simulink model "Sim_Multi"  (R2019b)
settings: Solver=VariableStepAuto  StartTime=0.0  StopTime=sim_time  FixedStep=t_sim  MaxStep=t_control  RelTol=1e-5  EnableMultiTasking=on
model workspace (MAT data in the model file):
  start_time = 1
values from neighbouring files (symbols this model uses):
  Att_init = [0;0;0] * d2r    [Init_Multi.m]
  Blade_flapping = 0    [Init_Multi.m]
  C_D = 0.40    (= 0.4)    [Init_Multi.m]
  CoG_nominal = [0;0;0.001]    [Init_Multi.m]
  CoG_real = [0;0;0.001]    [Init_Multi.m]
  Coriolis_correction = 0    [Init_Multi.m]
  d2r = pi/180    (= 0.0174532925199)    [Init_Multi.m]
  Dyn_thrust = 0    [Init_Multi.m]
  g = 9.80665    [Init_Multi.m]
  J_nominal = [Jxx Jxy Jxz;Jyx Jyy Jyz;Jzx Jzy Jzz]    [Init_Multi.m]
  J_real = [Jxx Jxy Jxz;Jyx Jyy Jyz;Jzx Jzy Jzz]    [Init_Multi.m]
  k1 = -1.125    [Init_Multi.m]
  k2 = -1.372    [Init_Multi.m]
  k3 = -1.718    [Init_Multi.m]
  k4 = -0.655    [Init_Multi.m]
  k_a1s = 1.5 / 4.0    (= 0.375)    [Init_Multi.m]
  k_beta = 0.23    [Init_Multi.m]
  kappa = 1.00    (= 1)    [Init_Multi.m]
  mass_nominal = 0.550    (= 0.55)    [Init_Multi.m]
  mass_real = 0.550    (= 0.55)    [Init_Multi.m]
  max_thrust = max_thrust + (MotorMatrix_nominal(i,7)*MotorMatrix_nominal(i,12)+MotorMatrix_nominal(i,8)*MotorMatrix_nominal(i,12)^2)    [Init_Multi.m]
  MaxRate_cmd = [360;360;120] * d2r    [Init_Multi.m]
  min_thrust = min_thrust + (MotorMatrix_nominal(i,7)*MotorMatrix_nominal(i,11)+MotorMatrix_nominal(i,8)*MotorMatrix_nominal(i,11)^2)    [Init_Multi.m]
  MotorMap = B' * inv(B * B')    [Init_Multi.m]
  MotorMatrix_nominal = [045 , 0.170 , -0.028 , -1 , 1.0 , 0.010 , [9.6820 , 0.010872]*1e-5 , [1.4504 , 0.0016312]*1e-6 , 0000 , 6000 , [0.0 , 0.0 , 0.0] , 8*2.54/100 , 11/1000;                         135 , 0.170 , -0.028 , +1 , 1.0 , 0.010 , [9.6820 , 0.010872]*1e-5 , [1.4504 , 0.0016312]*1e-6 , 0000 , 6000 , [0.0 , 0.0 , 0.0] , 8*2.54/100 , 11/1000;                         225 , 0.170 , -0.028 , -1 , 1.0 , 0.010 , [9. ...(+284 chars)    [Init_Multi.m]
  MotorMatrix_real = [045 , 0.170 , -0.028 , -1 , 1.0 , 0.010 , [9.6820 , 0.010872]*1e-5 , [1.4504 , 0.0016312]*1e-6 , 0000 , 6000 , [0.0 , 0.0 , 0.0] , 8*2.54/100 , 11/1000;                      135 , 0.170 , -0.028 , +1 , 1.0 , 0.010 , [9.6820 , 0.010872]*1e-5 , [1.4504 , 0.0016312]*1e-6 , 0000 , 6000 , [0.0 , 0.0 , 0.0] , 8*2.54/100 , 11/1000;                      225 , 0.170 , -0.028 , -1 , 1.0 , 0.010 , [9.6820 , ...(+275 chars)    [Init_Multi.m]
  Noise_flag = 1    [Init_Multi.m]
  omega_init = [0;0;0]    [Init_Multi.m]
  q_init = rpy2quat(Att_init)    [Init_Multi.m]
  r2d = 180/pi    (= 57.2957795131)    [Init_Multi.m]
  rho = 1.225    [Init_Multi.m]
  rpm2radpersec = 2*pi/60    (= 0.10471975512)    [Init_Multi.m]
  rpm_init = 3104.5025852    [Init_Multi.m]
  Surface_params = [a;b;c]    [Init_Multi.m]
  t_control = t_control_2*4    (= 0.02)    [Init_Multi.m]
  t_sim = 1/1000    (= 0.001)    [Init_Multi.m]
  thrust_reserve = 0.10    (= 0.1)    [Init_Multi.m]
  v_h = 4.0    (= 4)    [Init_Multi.m]
  Vb_init = [0;0;0]    [Init_Multi.m]
  Vi_init = R_IB_init' * Vb_init    [Init_Multi.m]
  Xi_init = [0;0;-1]    [Init_Multi.m]
undefined symbols (not defined in the file or in its folder): anti_windup_1, anti_windup_2, DiscIntNeverNeededParam, Kd_1, Kd_2, Kff_1, Kff_2, Ki_1, Ki_2, Kp_1, Kp_2, Kpass_1, magnitude, rpy2quat, thrust2rpm
libraries: simulink x35, dspsigops x3, sharedtransform x2, dspmtrx3 x1, robotuavlib x1, vrlib x1
(part 2 of 4)

== system Sim_Multi/State Estimation, Sensors, Noise/State estimation/Quat noise1 ==
  Band-Limited White Noise : simulink/Sources/Band-Limited White Noise  Cov=t_sim*57.3*57.3/10000  Ts=t_sim*30  seed=[23099]
  Constant : Constant  Value=Noise_flag
  Constant1 : Constant  Value=0
  Gain2 : Gain  Gain=0.1
  Rate Transition1 : RateTransition  OutPortSampleTime=t_sim
  Switch : Switch  Criteria=u2 > Threshold
  Noise : Outport
  wires:
  Band-Limited White Noise/1 -> Gain2/1
  Switch/1 -> Noise/1
  Constant/1 -> Switch/2
  Constant1/1 -> Switch/3
  Gain2/1 -> Rate Transition1/1
  Rate Transition1/1 -> Switch/1

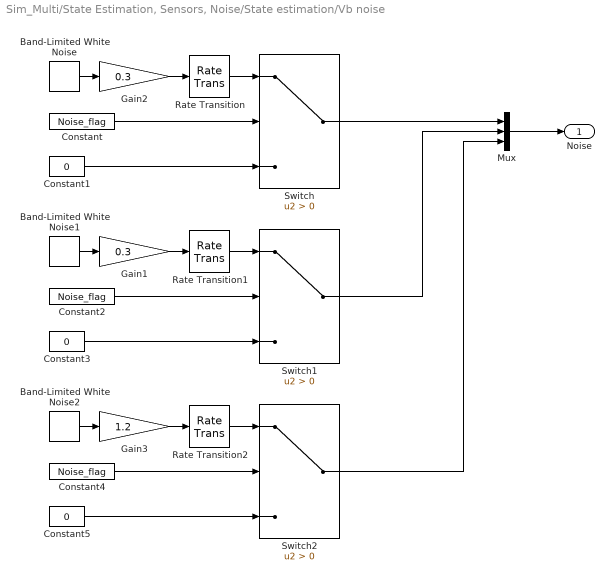
== system Sim_Multi/State Estimation, Sensors, Noise/State estimation/Vb noise ==
  Band-Limited White Noise : simulink/Sources/Band-Limited White Noise  Cov=t_sim*57.3*57.3/10000  Ts=t_sim*10  seed=[21234]
  Band-Limited White Noise1 : simulink/Sources/Band-Limited White Noise  Cov=t_sim*57.3*57.3/10000  Ts=t_sim*10  seed=[21234]
  Band-Limited White Noise2 : simulink/Sources/Band-Limited White Noise  Cov=t_sim*57.3*57.3/10000  Ts=t_sim*10  seed=[21234]
  Constant : Constant  Value=Noise_flag
  Constant1 : Constant  Value=0
  Constant2 : Constant  Value=Noise_flag
  Constant3 : Constant  Value=0
  Constant4 : Constant  Value=Noise_flag
  Constant5 : Constant  Value=0
  Gain1 : Gain  Gain=0.3
  Gain2 : Gain  Gain=0.3
  Gain3 : Gain  Gain=1.2
  Mux : Mux  Inputs=3
  Rate Transition : RateTransition  OutPortSampleTime=t_sim
  Rate Transition1 : RateTransition  OutPortSampleTime=t_sim
  Rate Transition2 : RateTransition  OutPortSampleTime=t_sim
  Switch : Switch  Criteria=u2 > Threshold
  Switch1 : Switch  Criteria=u2 > Threshold
  Switch2 : Switch  Criteria=u2 > Threshold
  Noise : Outport
  wires:
  Band-Limited White Noise/1 -> Gain2/1
  Constant/1 -> Switch/2
  Constant1/1 -> Switch/3
  Gain2/1 -> Rate Transition/1
  Rate Transition/1 -> Switch/1
  Switch/1 -> Mux/1
  Mux/1 -> Noise/1
  Band-Limited White Noise1/1 -> Gain1/1
  Constant2/1 -> Switch1/2
  Constant3/1 -> Switch1/3
  Gain1/1 -> Rate Transition1/1
  Rate Transition1/1 -> Switch1/1
  Band-Limited White Noise2/1 -> Gain3/1
  Constant4/1 -> Switch2/2
  Constant5/1 -> Switch2/3
  Gain3/1 -> Rate Transition2/1
  Rate Transition2/1 -> Switch2/1
  Switch1/1 -> Mux/2
  Switch2/1 -> Mux/3

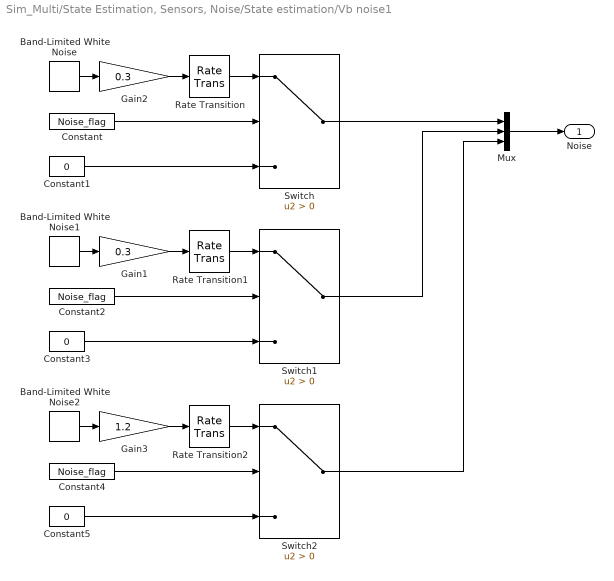
== system Sim_Multi/State Estimation, Sensors, Noise/State estimation/Vb noise1 ==
  Band-Limited White Noise : simulink/Sources/Band-Limited White Noise  Cov=t_sim*57.3*57.3/10000  Ts=t_sim*10  seed=[21234]
  Band-Limited White Noise1 : simulink/Sources/Band-Limited White Noise  Cov=t_sim*57.3*57.3/10000  Ts=t_sim*10  seed=[21234]
  Band-Limited White Noise2 : simulink/Sources/Band-Limited White Noise  Cov=t_sim*57.3*57.3/10000  Ts=t_sim*10  seed=[21234]
  Constant : Constant  Value=Noise_flag
  Constant1 : Constant  Value=0
  Constant2 : Constant  Value=Noise_flag
  Constant3 : Constant  Value=0
  Constant4 : Constant  Value=Noise_flag
  Constant5 : Constant  Value=0
  Gain1 : Gain  Gain=0.3
  Gain2 : Gain  Gain=0.3
  Gain3 : Gain  Gain=1.2
  Mux : Mux  Inputs=3
  Rate Transition : RateTransition  OutPortSampleTime=t_sim
  Rate Transition1 : RateTransition  OutPortSampleTime=t_sim
  Rate Transition2 : RateTransition  OutPortSampleTime=t_sim
  Switch : Switch  Criteria=u2 > Threshold
  Switch1 : Switch  Criteria=u2 > Threshold
  Switch2 : Switch  Criteria=u2 > Threshold
  Noise : Outport
  wires:
  Band-Limited White Noise/1 -> Gain2/1
  Constant/1 -> Switch/2
  Constant1/1 -> Switch/3
  Gain2/1 -> Rate Transition/1
  Rate Transition/1 -> Switch/1
  Switch/1 -> Mux/1
  Mux/1 -> Noise/1
  Band-Limited White Noise1/1 -> Gain1/1
  Constant2/1 -> Switch1/2
  Constant3/1 -> Switch1/3
  Gain1/1 -> Rate Transition1/1
  Rate Transition1/1 -> Switch1/1
  Band-Limited White Noise2/1 -> Gain3/1
  Constant4/1 -> Switch2/2
  Constant5/1 -> Switch2/3
  Gain3/1 -> Rate Transition2/1
  Rate Transition2/1 -> Switch2/1
  Switch1/1 -> Mux/2
  Switch2/1 -> Mux/3

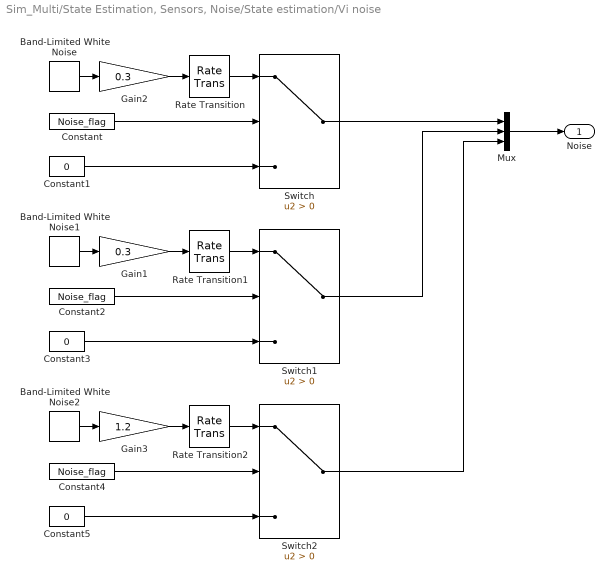
== system Sim_Multi/State Estimation, Sensors, Noise/State estimation/Vi noise ==
  Band-Limited White Noise : simulink/Sources/Band-Limited White Noise  Cov=t_sim*57.3*57.3/10000  Ts=t_sim*10  seed=[23888]
  Band-Limited White Noise1 : simulink/Sources/Band-Limited White Noise  Cov=t_sim*57.3*57.3/10000  Ts=t_sim*10  seed=[23888]
  Band-Limited White Noise2 : simulink/Sources/Band-Limited White Noise  Cov=t_sim*57.3*57.3/10000  Ts=t_sim*10  seed=[23888]
  Constant : Constant  Value=Noise_flag
  Constant1 : Constant  Value=0
  Constant2 : Constant  Value=Noise_flag
  Constant3 : Constant  Value=0
  Constant4 : Constant  Value=Noise_flag
  Constant5 : Constant  Value=0
  Gain1 : Gain  Gain=0.3
  Gain2 : Gain  Gain=0.3
  Gain3 : Gain  Gain=1.2
  Mux : Mux  Inputs=3
  Rate Transition : RateTransition  OutPortSampleTime=t_sim
  Rate Transition1 : RateTransition  OutPortSampleTime=t_sim
  Rate Transition2 : RateTransition  OutPortSampleTime=t_sim
  Switch : Switch  Criteria=u2 > Threshold
  Switch1 : Switch  Criteria=u2 > Threshold
  Switch2 : Switch  Criteria=u2 > Threshold
  Noise : Outport
  wires:
  Band-Limited White Noise/1 -> Gain2/1
  Constant/1 -> Switch/2
  Constant1/1 -> Switch/3
  Gain2/1 -> Rate Transition/1
  Rate Transition/1 -> Switch/1
  Switch/1 -> Mux/1
  Mux/1 -> Noise/1
  Band-Limited White Noise1/1 -> Gain1/1
  Constant2/1 -> Switch1/2
  Constant3/1 -> Switch1/3
  Gain1/1 -> Rate Transition1/1
  Rate Transition1/1 -> Switch1/1
  Band-Limited White Noise2/1 -> Gain3/1
  Constant4/1 -> Switch2/2
  Constant5/1 -> Switch2/3
  Gain3/1 -> Rate Transition2/1
  Rate Transition2/1 -> Switch2/1
  Switch1/1 -> Mux/2
  Switch2/1 -> Mux/3

== system Sim_Multi/State Estimation, Sensors, Noise/State estimation/Vi noise1 ==
  Band-Limited White Noise : simulink/Sources/Band-Limited White Noise  Cov=t_sim*57.3*57.3/10000  Ts=t_sim*10  seed=[23888]
  Band-Limited White Noise1 : simulink/Sources/Band-Limited White Noise  Cov=t_sim*57.3*57.3/10000  Ts=t_sim*10  seed=[23888]
  Band-Limited White Noise2 : simulink/Sources/Band-Limited White Noise  Cov=t_sim*57.3*57.3/10000  Ts=t_sim*10  seed=[23888]
  Constant : Constant  Value=Noise_flag
  Constant1 : Constant  Value=0
  Constant2 : Constant  Value=Noise_flag
  Constant3 : Constant  Value=0
  Constant4 : Constant  Value=Noise_flag
  Constant5 : Constant  Value=0
  Gain1 : Gain  Gain=0.3
  Gain2 : Gain  Gain=0.3
  Gain3 : Gain  Gain=1.2
  Mux : Mux  Inputs=3
  Rate Transition : RateTransition  OutPortSampleTime=t_sim
  Rate Transition1 : RateTransition  OutPortSampleTime=t_sim
  Rate Transition2 : RateTransition  OutPortSampleTime=t_sim
  Switch : Switch  Criteria=u2 > Threshold
  Switch1 : Switch  Criteria=u2 > Threshold
  Switch2 : Switch  Criteria=u2 > Threshold
  Noise : Outport
  wires:
  Band-Limited White Noise/1 -> Gain2/1
  Constant/1 -> Switch/2
  Constant1/1 -> Switch/3
  Gain2/1 -> Rate Transition/1
  Rate Transition/1 -> Switch/1
  Switch/1 -> Mux/1
  Mux/1 -> Noise/1
  Band-Limited White Noise1/1 -> Gain1/1
  Constant2/1 -> Switch1/2
  Constant3/1 -> Switch1/3
  Gain1/1 -> Rate Transition1/1
  Rate Transition1/1 -> Switch1/1
  Band-Limited White Noise2/1 -> Gain3/1
  Constant4/1 -> Switch2/2
  Constant5/1 -> Switch2/3
  Gain3/1 -> Rate Transition2/1
  Rate Transition2/1 -> Switch2/1
  Switch1/1 -> Mux/2
  Switch2/1 -> Mux/3

== system Sim_Multi/State Estimation, Sensors, Noise/State estimation/Xi noise ==
  Band-Limited White Noise : simulink/Sources/Band-Limited White Noise  Cov=t_sim*57.3*57.3/10000  Ts=t_sim*20  seed=[23559]
  Band-Limited White Noise1 : simulink/Sources/Band-Limited White Noise  Cov=t_sim*57.3*57.3/10000  Ts=t_sim*20  seed=[23559]
  Band-Limited White Noise2 : simulink/Sources/Band-Limited White Noise  Cov=t_sim*57.3*57.3/10000  Ts=t_sim*20  seed=[23559]
  Constant : Constant  Value=Noise_flag
  Constant1 : Constant  Value=0
  Constant2 : Constant  Value=Noise_flag
  Constant3 : Constant  Value=0
  Constant4 : Constant  Value=Noise_flag
  Constant5 : Constant  Value=0
  Gain1 : Gain  Gain=0.1
  Gain2 : Gain  Gain=0.1
  Gain3 : Gain  Gain=0.7
  Mux : Mux  Inputs=3
  Rate Transition : RateTransition  OutPortSampleTime=t_sim
  Rate Transition1 : RateTransition  OutPortSampleTime=t_sim
  Rate Transition2 : RateTransition  OutPortSampleTime=t_sim
  Switch : Switch  Criteria=u2 > Threshold
  Switch1 : Switch  Criteria=u2 > Threshold
  Switch2 : Switch  Criteria=u2 > Threshold
  Noise : Outport
  wires:
  Band-Limited White Noise/1 -> Gain2/1
  Constant/1 -> Switch/2
  Constant1/1 -> Switch/3
  Gain2/1 -> Rate Transition/1
  Mux/1 -> Noise/1
  Switch/1 -> Mux/1
  Band-Limited White Noise1/1 -> Gain1/1
  Constant2/1 -> Switch1/2
  Constant3/1 -> Switch1/3
  Gain1/1 -> Rate Transition1/1
  Band-Limited White Noise2/1 -> Gain3/1
  Constant4/1 -> Switch2/2
  Constant5/1 -> Switch2/3
  Gain3/1 -> Rate Transition2/1
  Switch1/1 -> Mux/2
  Switch2/1 -> Mux/3
  Rate Transition/1 -> Switch/1
  Rate Transition1/1 -> Switch1/1
  Rate Transition2/1 -> Switch2/1

== system Sim_Multi/State Estimation, Sensors, Noise/State estimation/Xi noise1 ==
  Band-Limited White Noise : simulink/Sources/Band-Limited White Noise  Cov=t_sim*57.3*57.3/10000  Ts=t_sim*20  seed=[23559]
  Band-Limited White Noise1 : simulink/Sources/Band-Limited White Noise  Cov=t_sim*57.3*57.3/10000  Ts=t_sim*20  seed=[23559]
  Band-Limited White Noise2 : simulink/Sources/Band-Limited White Noise  Cov=t_sim*57.3*57.3/10000  Ts=t_sim*20  seed=[23559]
  Constant : Constant  Value=Noise_flag
  Constant1 : Constant  Value=0
  Constant2 : Constant  Value=Noise_flag
  Constant3 : Constant  Value=0
  Constant4 : Constant  Value=Noise_flag
  Constant5 : Constant  Value=0
  Gain1 : Gain  Gain=0.1
  Gain2 : Gain  Gain=0.1
  Gain3 : Gain  Gain=0.7
  Mux : Mux  Inputs=3
  Rate Transition : RateTransition  OutPortSampleTime=t_sim
  Rate Transition1 : RateTransition  OutPortSampleTime=t_sim
  Rate Transition2 : RateTransition  OutPortSampleTime=t_sim
  Switch : Switch  Criteria=u2 > Threshold
  Switch1 : Switch  Criteria=u2 > Threshold
  Switch2 : Switch  Criteria=u2 > Threshold
  Noise : Outport
  wires:
  Band-Limited White Noise/1 -> Gain2/1
  Constant/1 -> Switch/2
  Constant1/1 -> Switch/3
  Gain2/1 -> Rate Transition/1
  Mux/1 -> Noise/1
  Switch/1 -> Mux/1
  Band-Limited White Noise1/1 -> Gain1/1
  Constant2/1 -> Switch1/2
  Constant3/1 -> Switch1/3
  Gain1/1 -> Rate Transition1/1
  Band-Limited White Noise2/1 -> Gain3/1
  Constant4/1 -> Switch2/2
  Constant5/1 -> Switch2/3
  Gain3/1 -> Rate Transition2/1
  Switch1/1 -> Mux/2
  Switch2/1 -> Mux/3
  Rate Transition/1 -> Switch/1
  Rate Transition1/1 -> Switch1/1
  Rate Transition2/1 -> Switch2/1

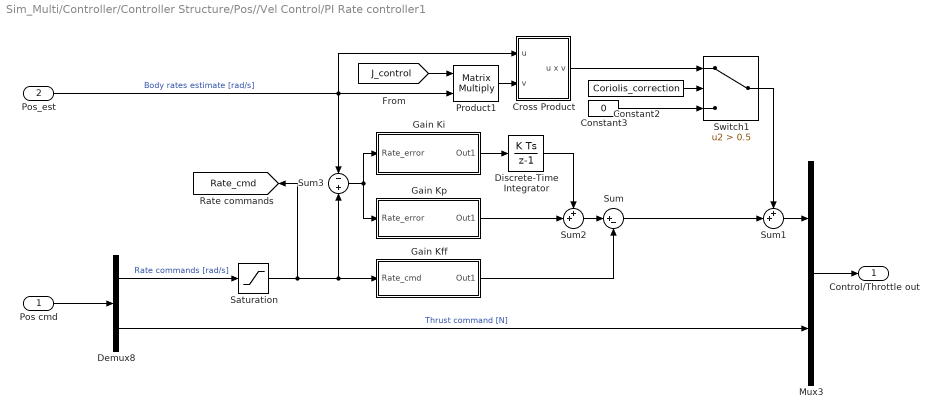
== system Sim_Multi/Controller/Controller Structure/Pos//Vel Control/PI Rate controller1 ==
  Pos cmd : Inport
  Pos_est : Inport  Port=2
  Constant2 : Constant  Value=Coriolis_correction
  Constant3 : Constant  Value=0
  Cross Product : Subsystem
  Demux8 : Demux  Outputs=[3 1]
  Discrete-Time Integrator : DiscreteIntegrator  SampleTime=t_control  ICPrevOutput=DiscIntNeverNeededParam  ICPrevScaledInput=DiscIntNeverNeededParam
  Gain Kff : Subsystem
  Gain Ki : Subsystem
  Gain Kp : Subsystem
  Mux3 : Mux  Inputs=2
  Product1 : Product  Multiplication=Matrix(*)  SampleTime=t_control  RndMeth=Zero
  Saturation : Saturate  UpperLimit=MaxRate_cmd  LowerLimit=-MaxRate_cmd
  Sum : Sum  Inputs=|+-
  Sum1 : Sum  Inputs=++|
  Sum2 : Sum  Inputs=++|
  Sum3 : Sum  Inputs=-|+
  Switch1 : Switch  Criteria=u2 > Threshold  Threshold=0.5  SampleTime=t_control
  Control/Throttle out : Outport
  tag scope: Rate_cmd=global
  wires:
  Pos_est/1 -> Product1/2, Sum3/1, Cross Product/1(u)  "Body rates estimate [rad/s]"
  Mux3/1 -> Control/Throttle out/1
  Pos cmd/1 -> Demux8/1
  Gain Ki/1(Out1) -> Discrete-Time Integrator/1
  Discrete-Time Integrator/1 -> Sum2/1
  Gain Kp/1(Out1) -> Sum2/2
  [J_control] -> Product1/1
  Product1/1 -> Cross Product/2(v)
  Sum1/1 -> Mux3/1
  Demux8/1 -> Saturation/1  "Rate commands [rad/s]"
  Sum3/1 -> Gain Kp/1(Rate_error), Gain Ki/1(Rate_error)
  Sum/1 -> Sum1/2
  Sum2/1 -> Sum/1
  Gain Kff/1(Out1) -> Sum/2
  Demux8/2 -> Mux3/2  "Thrust command [N]"
  Constant2/1 -> Switch1/2
  Cross Product/1(u x v) -> Switch1/1
  Constant3/1 -> Switch1/3
  Switch1/1 -> Sum1/1
  Saturation/1 -> [Rate_cmd], Sum3/2, Gain Kff/1(Rate_cmd)

== system Sim_Multi/Controller/Controller Structure/Pos//Vel Control/PID Attitude Controller (additionally controls altitude and yaw to take advantage of faster sampling rate)1 ==
  roll,pitch,yaw,Z_cmd : Inport
  roll,pitch,yaw,Z_est : Inport  Port=2
  Commands : Goto  Commented=on  GotoTag=rate_cmd  TagVisibility=global
  Constant : Constant  Value=Kff_2  SampleTime=-1
  Discrete Derivative : simulink/Discrete/Discrete Derivative  gainval=1.0  ICPrevScaledInput=0.0  OutMin=[]  OutMax=[]  OutDataType=fixdt(1, 16)  OutScaling=2^-10  DoSatur=off
  Discrete-Time Integrator : DiscreteIntegrator  SampleTime=-1  LimitOutput=on  UpperSaturationLimit=anti_windup_2  LowerSaturationLimit=-1*anti_windup_2  ICPrevOutput=DiscIntNeverNeededParam  ICPrevScaledInput=DiscIntNeverNeededParam
  Gain Kd : Subsystem
  Gain Ki : Subsystem
  Gain Kp : Subsystem
  Rate Transition : RateTransition  OutPortSampleTime=t_control_2
  Rate Transition1 : RateTransition  OutPortSampleTime=t_control_2
  Sum : Sum  Inputs=+++
  Sum2 : Sum  Inputs=++|
  Sum3 : Sum  Inputs=-|+
  Control/Velocity out : Outport
  wires:
  roll,pitch,yaw,Z_est/1 -> Rate Transition/1  "Body rates estimate [rad/s]"
  Sum/1 -> Control/Velocity out/1
  Gain Ki/1(Out1) -> Discrete-Time Integrator/1
  Discrete-Time Integrator/1 -> Sum2/1
  Gain Kp/1(Out1) -> Sum2/2
  Sum3/1 -> Gain Kp/1(Rate_error), Gain Ki/1(Rate_error)
  roll,pitch,yaw,Z_cmd/1 -> Rate Transition1/1
  Gain Kd/1(Out1) -> Sum/1
  Sum2/1 -> Sum/2
  Constant/1 -> Sum/3
  Discrete Derivative/1 -> Gain Kd/1(Rate_error)
  Rate Transition/1 -> Discrete Derivative/1, Sum3/1
  Rate Transition1/1 -> Commands/1, Sum3/2

== system Sim_Multi/Controller/Controller Structure/Pos//Vel Control/PID Attitude//Altitude Contorller ==
  roll,pitch,yaw,Z_cmd : Inport
  roll,pitch,yaw,Z_est : Inport  Port=2
  Constant : Constant  Value=5.4
  Demux : Demux
  Gain{,1..3} (4 alike) : Gain
  Mux : Mux
  PID Controller1 : simulink/Continuous/PID Controller  Controller=PID  Form=Parallel  TimeDomain=Discrete-time  SampleTime=-1  IntegratorMethod=Forward Euler  FilterMethod=Forward Euler  ControllerParametersSource=internal  P=0.061831432569432  I=0.0240439713230998  D=0.0379888953879029  UseFilter=on  N=83.1174994512611  TunerSelectOption=Transfer Function Based (PID Tuner App)  InitialConditionSource=internal  InitialConditionForIntegrator=0  InitialConditionForFilter=0  DifferentiatorICPrevScaledInput=0  ExternalReset=none  TrackingMode=off  Kt=1  LimitOutput=off  UpperSaturationLimit=inf  LowerSaturationLimit=-inf  LinearizeAsGain=on  AntiWindupMode=none  Kb=1  POutMin=[]  POutMax=[]  IOutMin=[]  IOutMax=[]  DOutMin=[]  DOutMax=[]  NOutMin=[]  NOutMax=[]  SumOutMin=[]  SumOutMax=[]  SaturationOutMin=[]  SaturationOutMax=[]  PParamMin=[]  PParamMax=[]  IParamMin=[]  IParamMax=[]  DParamMin=[]  DParamMax=[]  NParamMin=[]  NParamMax=[]  KbParamMin=[]  KbParamMax=[]  KtParamMin=[]  KtParamMax=[]  KbOutMin=[]  KbOutMax=[]  KtOutMin=[]  KtOutMax=[]  IntegratorOutMin=[]  IntegratorOutMax=[]  FilterOutMin=[]  FilterOutMax=[]  SumI1OutMin=[]  SumI1OutMax=[]  SumI2OutMin=[]  SumI2OutMax=[]  SumI3OutMin=[]  SumI3OutMax=[]  SumI4OutMin=[]  SumI4OutMax=[]  SumDOutMin=[]  SumDOutMax=[]  DifferentiatorOutMin=[]  DifferentiatorOutMax=[]  FilterDiffOutCoefMin=[]  FilterDiffOutCoefMax=[]  ReciprocalOutMin=[]  ReciprocalOutMax=[]  SumDenOutMin=[]  SumDenOutMax=[]  SumNumOutMin=[]  SumNumOutMax=[]  DivideOutMin=[]  DivideOutMax=[]  IntegratorContinuousStateAttributes=''  IntegratorStateMustResolveToSignalObject=off  IntegratorRTWStateStorageClass=Auto  FilterContinuousStateAttributes=''  FilterStateMustResolveToSignalObject=off  FilterRTWStateStorageClass=Auto  ParallelPVariant=InternalParameters  IdealPVariant=Disabled  IVariant=InternalParameters  DVariant=InternalParameters  IntegratorVariant=Discrete  SatVariant=Disabled  AWVariant=Passthrough  PCopyVariant=Disabled  TRVariant=Disabled  FdbkBlocksVariant=Forward  IdealPFdbkVariant=Disabled  SatFdbkVariant=Disabled  DerivativeFilterVariant=ForwardEulerFilter  NVariant=InternalParameters  NCopyVariant=Disabled  FilterICVariant=InternalICsFilter  IntegratorICVariant=InternalICs  ExternalResetVariant=Disabled  TRSumVariant=Passthrough  SumFdbkVariant=Disabled  SumVariant=Sum_PID
  PID Controller2 : simulink/Continuous/PID Controller  Controller=PID  Form=Parallel  TimeDomain=Discrete-time  SampleTime=-1  IntegratorMethod=Forward Euler  FilterMethod=Forward Euler  ControllerParametersSource=internal  P=0.00183714357509643  I=9.47923809923689e-05  D=0.00707292143048776  UseFilter=on  N=10.221680571317  TunerSelectOption=Transfer Function Based (PID Tuner App)  InitialConditionSource=internal  InitialConditionForIntegrator=0  InitialConditionForFilter=0  DifferentiatorICPrevScaledInput=0  ExternalReset=none  TrackingMode=off  Kt=1  LimitOutput=off  UpperSaturationLimit=inf  LowerSaturationLimit=-inf  LinearizeAsGain=on  AntiWindupMode=none  Kb=1  POutMin=[]  POutMax=[]  IOutMin=[]  IOutMax=[]  DOutMin=[]  DOutMax=[]  NOutMin=[]  NOutMax=[]  SumOutMin=[]  SumOutMax=[]  SaturationOutMin=[]  SaturationOutMax=[]  PParamMin=[]  PParamMax=[]  IParamMin=[]  IParamMax=[]  DParamMin=[]  DParamMax=[]  NParamMin=[]  NParamMax=[]  KbParamMin=[]  KbParamMax=[]  KtParamMin=[]  KtParamMax=[]  KbOutMin=[]  KbOutMax=[]  KtOutMin=[]  KtOutMax=[]  IntegratorOutMin=[]  IntegratorOutMax=[]  FilterOutMin=[]  FilterOutMax=[]  SumI1OutMin=[]  SumI1OutMax=[]  SumI2OutMin=[]  SumI2OutMax=[]  SumI3OutMin=[]  SumI3OutMax=[]  SumI4OutMin=[]  SumI4OutMax=[]  SumDOutMin=[]  SumDOutMax=[]  DifferentiatorOutMin=[]  DifferentiatorOutMax=[]  FilterDiffOutCoefMin=[]  FilterDiffOutCoefMax=[]  ReciprocalOutMin=[]  ReciprocalOutMax=[]  SumDenOutMin=[]  SumDenOutMax=[]  SumNumOutMin=[]  SumNumOutMax=[]  DivideOutMin=[]  DivideOutMax=[]  IntegratorContinuousStateAttributes=''  IntegratorStateMustResolveToSignalObject=off  IntegratorRTWStateStorageClass=Auto  FilterContinuousStateAttributes=''  FilterStateMustResolveToSignalObject=off  FilterRTWStateStorageClass=Auto  ParallelPVariant=InternalParameters  IdealPVariant=Disabled  IVariant=InternalParameters  DVariant=InternalParameters  IntegratorVariant=Discrete  SatVariant=Disabled  AWVariant=Passthrough  PCopyVariant=Disabled  TRVariant=Disabled  FdbkBlocksVariant=Forward  IdealPFdbkVariant=Disabled  SatFdbkVariant=Disabled  DerivativeFilterVariant=ForwardEulerFilter  NVariant=InternalParameters  NCopyVariant=Disabled  FilterICVariant=InternalICsFilter  IntegratorICVariant=InternalICs  ExternalResetVariant=Disabled  TRSumVariant=Passthrough  SumFdbkVariant=Disabled  SumVariant=Sum_PID
  PID Controller3 : simulink/Continuous/PID Controller  Controller=PID  Form=Parallel  TimeDomain=Discrete-time  SampleTime=-1  IntegratorMethod=Forward Euler  FilterMethod=Forward Euler  ControllerParametersSource=internal  P=-0.137480258273751  I=-0.00709366496874399  D=-0.529292907856896  UseFilter=on  N=10.221680571317  TunerSelectOption=Transfer Function Based (PID Tuner App)  InitialConditionSource=internal  InitialConditionForIntegrator=0  InitialConditionForFilter=0  DifferentiatorICPrevScaledInput=0  ExternalReset=none  TrackingMode=off  Kt=1  LimitOutput=off  UpperSaturationLimit=inf  LowerSaturationLimit=-inf  LinearizeAsGain=on  AntiWindupMode=none  Kb=1  POutMin=[]  POutMax=[]  IOutMin=[]  IOutMax=[]  DOutMin=[]  DOutMax=[]  NOutMin=[]  NOutMax=[]  SumOutMin=[]  SumOutMax=[]  SaturationOutMin=[]  SaturationOutMax=[]  PParamMin=[]  PParamMax=[]  IParamMin=[]  IParamMax=[]  DParamMin=[]  DParamMax=[]  NParamMin=[]  NParamMax=[]  KbParamMin=[]  KbParamMax=[]  KtParamMin=[]  KtParamMax=[]  KbOutMin=[]  KbOutMax=[]  KtOutMin=[]  KtOutMax=[]  IntegratorOutMin=[]  IntegratorOutMax=[]  FilterOutMin=[]  FilterOutMax=[]  SumI1OutMin=[]  SumI1OutMax=[]  SumI2OutMin=[]  SumI2OutMax=[]  SumI3OutMin=[]  SumI3OutMax=[]  SumI4OutMin=[]  SumI4OutMax=[]  SumDOutMin=[]  SumDOutMax=[]  DifferentiatorOutMin=[]  DifferentiatorOutMax=[]  FilterDiffOutCoefMin=[]  FilterDiffOutCoefMax=[]  ReciprocalOutMin=[]  ReciprocalOutMax=[]  SumDenOutMin=[]  SumDenOutMax=[]  SumNumOutMin=[]  SumNumOutMax=[]  DivideOutMin=[]  DivideOutMax=[]  IntegratorContinuousStateAttributes=''  IntegratorStateMustResolveToSignalObject=off  IntegratorRTWStateStorageClass=Auto  FilterContinuousStateAttributes=''  FilterStateMustResolveToSignalObject=off  FilterRTWStateStorageClass=Auto  ParallelPVariant=InternalParameters  IdealPVariant=Disabled  IVariant=InternalParameters  DVariant=InternalParameters  IntegratorVariant=Discrete  SatVariant=Disabled  AWVariant=Passthrough  PCopyVariant=Disabled  TRVariant=Disabled  FdbkBlocksVariant=Forward  IdealPFdbkVariant=Disabled  SatFdbkVariant=Disabled  DerivativeFilterVariant=ForwardEulerFilter  NVariant=InternalParameters  NCopyVariant=Disabled  FilterICVariant=InternalICsFilter  IntegratorICVariant=InternalICs  ExternalResetVariant=Disabled  TRSumVariant=Passthrough  SumFdbkVariant=Disabled  SumVariant=Sum_PID
  PID Controller4 : simulink/Continuous/PID Controller  Controller=PID  Form=Parallel  TimeDomain=Discrete-time  SampleTime=-1  IntegratorMethod=Forward Euler  FilterMethod=Forward Euler  ControllerParametersSource=internal  P=0.0636807472008284  I=0.0247631018062204  D=0.0391251042246079  UseFilter=on  N=83.1174994512611  TunerSelectOption=Transfer Function Based (PID Tuner App)  InitialConditionSource=internal  InitialConditionForIntegrator=0  InitialConditionForFilter=0  DifferentiatorICPrevScaledInput=0  ExternalReset=none  TrackingMode=off  Kt=1  LimitOutput=off  UpperSaturationLimit=inf  LowerSaturationLimit=-inf  LinearizeAsGain=on  AntiWindupMode=none  Kb=1  POutMin=[]  POutMax=[]  IOutMin=[]  IOutMax=[]  DOutMin=[]  DOutMax=[]  NOutMin=[]  NOutMax=[]  SumOutMin=[]  SumOutMax=[]  SaturationOutMin=[]  SaturationOutMax=[]  PParamMin=[]  PParamMax=[]  IParamMin=[]  IParamMax=[]  DParamMin=[]  DParamMax=[]  NParamMin=[]  NParamMax=[]  KbParamMin=[]  KbParamMax=[]  KtParamMin=[]  KtParamMax=[]  KbOutMin=[]  KbOutMax=[]  KtOutMin=[]  KtOutMax=[]  IntegratorOutMin=[]  IntegratorOutMax=[]  FilterOutMin=[]  FilterOutMax=[]  SumI1OutMin=[]  SumI1OutMax=[]  SumI2OutMin=[]  SumI2OutMax=[]  SumI3OutMin=[]  SumI3OutMax=[]  SumI4OutMin=[]  SumI4OutMax=[]  SumDOutMin=[]  SumDOutMax=[]  DifferentiatorOutMin=[]  DifferentiatorOutMax=[]  FilterDiffOutCoefMin=[]  FilterDiffOutCoefMax=[]  ReciprocalOutMin=[]  ReciprocalOutMax=[]  SumDenOutMin=[]  SumDenOutMax=[]  SumNumOutMin=[]  SumNumOutMax=[]  DivideOutMin=[]  DivideOutMax=[]  IntegratorContinuousStateAttributes=''  IntegratorStateMustResolveToSignalObject=off  IntegratorRTWStateStorageClass=Auto  FilterContinuousStateAttributes=''  FilterStateMustResolveToSignalObject=off  FilterRTWStateStorageClass=Auto  ParallelPVariant=InternalParameters  IdealPVariant=Disabled  IVariant=InternalParameters  DVariant=InternalParameters  IntegratorVariant=Discrete  SatVariant=Disabled  AWVariant=Passthrough  PCopyVariant=Disabled  TRVariant=Disabled  FdbkBlocksVariant=Forward  IdealPFdbkVariant=Disabled  SatFdbkVariant=Disabled  DerivativeFilterVariant=ForwardEulerFilter  NVariant=InternalParameters  NCopyVariant=Disabled  FilterICVariant=InternalICsFilter  IntegratorICVariant=InternalICs  ExternalResetVariant=Disabled  TRSumVariant=Passthrough  SumFdbkVariant=Disabled  SumVariant=Sum_PID
  Rate Transition1 : RateTransition  OutPortSampleTime=t_control_2
  Rate Transition2 : RateTransition  OutPortSampleTime=t_control_2
  Scope3 : Scope  NumInputPorts=4
  Sum : Sum  Inputs=|++
  Sum3 : Sum  Inputs=-|+
  Control/Velocity out : Outport
  wires:
  PID Controller3/1 -> Gain3/1
  PID Controller1/1 -> Gain1/1
  Gain/1 -> Mux/1
  roll,pitch,yaw,Z_cmd/1 -> Rate Transition1/1
  Gain2/1 -> Mux/3
  Sum3/1 -> Demux/1
  Mux/1 -> Rate Transition2/1
  Sum/1 -> Mux/4
  PID Controller2/1 -> Gain2/1
  Gain3/1 -> Sum/1
  Constant/1 -> Sum/2
  PID Controller4/1 -> Gain/1
  roll,pitch,yaw,Z_est/1 -> Sum3/1
  Gain1/1 -> Mux/2
  Demux/2 -> Scope3/2, PID Controller1/1
  Rate Transition1/1 -> Sum3/2
  Demux/4 -> Scope3/4, PID Controller3/1
  Demux/3 -> Scope3/3, PID Controller2/1
  Demux/1 -> Scope3/1, PID Controller4/1
  Rate Transition2/1 -> Control/Velocity out/1

== system Sim_Multi/Controller/Controller Structure/Pos//Vel Control/PID Position Controller (yaw and Z are passed though) ==
  (Y,X,yaw,Z)_cmd : Inport
  (Y,X,yaw,Z)_est : Inport  Port=2
  Demux : Demux
  Demux1 : Demux
  Gain : Gain
  Gain1 : Gain
  Mux : Mux
  PID Controller1 : simulink/Continuous/PID Controller  Controller=PID  Form=Parallel  TimeDomain=Discrete-time  SampleTime=-1  IntegratorMethod=Forward Euler  FilterMethod=Forward Euler  ControllerParametersSource=internal  P=-0.0202827380782485  I=-0.00081616740602595  D=-0.0881024693027783  UseFilter=on  N=9.03936793379723  TunerSelectOption=Transfer Function Based (PID Tuner App)  InitialConditionSource=internal  InitialConditionForIntegrator=0  InitialConditionForFilter=0  DifferentiatorICPrevScaledInput=0  ExternalReset=none  TrackingMode=off  Kt=1  LimitOutput=off  UpperSaturationLimit=inf  LowerSaturationLimit=-inf  LinearizeAsGain=on  AntiWindupMode=none  Kb=1  POutMin=[]  POutMax=[]  IOutMin=[]  IOutMax=[]  DOutMin=[]  DOutMax=[]  NOutMin=[]  NOutMax=[]  SumOutMin=[]  SumOutMax=[]  SaturationOutMin=[]  SaturationOutMax=[]  PParamMin=[]  PParamMax=[]  IParamMin=[]  IParamMax=[]  DParamMin=[]  DParamMax=[]  NParamMin=[]  NParamMax=[]  KbParamMin=[]  KbParamMax=[]  KtParamMin=[]  KtParamMax=[]  KbOutMin=[]  KbOutMax=[]  KtOutMin=[]  KtOutMax=[]  IntegratorOutMin=[]  IntegratorOutMax=[]  FilterOutMin=[]  FilterOutMax=[]  SumI1OutMin=[]  SumI1OutMax=[]  SumI2OutMin=[]  SumI2OutMax=[]  SumI3OutMin=[]  SumI3OutMax=[]  SumI4OutMin=[]  SumI4OutMax=[]  SumDOutMin=[]  SumDOutMax=[]  DifferentiatorOutMin=[]  DifferentiatorOutMax=[]  FilterDiffOutCoefMin=[]  FilterDiffOutCoefMax=[]  ReciprocalOutMin=[]  ReciprocalOutMax=[]  SumDenOutMin=[]  SumDenOutMax=[]  SumNumOutMin=[]  SumNumOutMax=[]  DivideOutMin=[]  DivideOutMax=[]  IntegratorContinuousStateAttributes=''  IntegratorStateMustResolveToSignalObject=off  IntegratorRTWStateStorageClass=Auto  FilterContinuousStateAttributes=''  FilterStateMustResolveToSignalObject=off  FilterRTWStateStorageClass=Auto  ParallelPVariant=InternalParameters  IdealPVariant=Disabled  IVariant=InternalParameters  DVariant=InternalParameters  IntegratorVariant=Discrete  SatVariant=Disabled  AWVariant=Passthrough  PCopyVariant=Disabled  TRVariant=Disabled  FdbkBlocksVariant=Forward  IdealPFdbkVariant=Disabled  SatFdbkVariant=Disabled  DerivativeFilterVariant=ForwardEulerFilter  NVariant=InternalParameters  NCopyVariant=Disabled  FilterICVariant=InternalICsFilter  IntegratorICVariant=InternalICs  ExternalResetVariant=Disabled  TRSumVariant=Passthrough  SumFdbkVariant=Disabled  SumVariant=Sum_PID
  PID Controller4 : simulink/Continuous/PID Controller  Controller=PID  Form=Parallel  TimeDomain=Discrete-time  SampleTime=-1  IntegratorMethod=Forward Euler  FilterMethod=Forward Euler  ControllerParametersSource=internal  P=0.0202827380772714  I=0.000816167405912946  D=0.0881024692983823  UseFilter=on  N=9.03936793379723  TunerSelectOption=Transfer Function Based (PID Tuner App)  InitialConditionSource=internal  InitialConditionForIntegrator=0  InitialConditionForFilter=0  DifferentiatorICPrevScaledInput=0  ExternalReset=none  TrackingMode=off  Kt=1  LimitOutput=off  UpperSaturationLimit=inf  LowerSaturationLimit=-inf  LinearizeAsGain=on  AntiWindupMode=none  Kb=1  POutMin=[]  POutMax=[]  IOutMin=[]  IOutMax=[]  DOutMin=[]  DOutMax=[]  NOutMin=[]  NOutMax=[]  SumOutMin=[]  SumOutMax=[]  SaturationOutMin=[]  SaturationOutMax=[]  PParamMin=[]  PParamMax=[]  IParamMin=[]  IParamMax=[]  DParamMin=[]  DParamMax=[]  NParamMin=[]  NParamMax=[]  KbParamMin=[]  KbParamMax=[]  KtParamMin=[]  KtParamMax=[]  KbOutMin=[]  KbOutMax=[]  KtOutMin=[]  KtOutMax=[]  IntegratorOutMin=[]  IntegratorOutMax=[]  FilterOutMin=[]  FilterOutMax=[]  SumI1OutMin=[]  SumI1OutMax=[]  SumI2OutMin=[]  SumI2OutMax=[]  SumI3OutMin=[]  SumI3OutMax=[]  SumI4OutMin=[]  SumI4OutMax=[]  SumDOutMin=[]  SumDOutMax=[]  DifferentiatorOutMin=[]  DifferentiatorOutMax=[]  FilterDiffOutCoefMin=[]  FilterDiffOutCoefMax=[]  ReciprocalOutMin=[]  ReciprocalOutMax=[]  SumDenOutMin=[]  SumDenOutMax=[]  SumNumOutMin=[]  SumNumOutMax=[]  DivideOutMin=[]  DivideOutMax=[]  IntegratorContinuousStateAttributes=''  IntegratorStateMustResolveToSignalObject=off  IntegratorRTWStateStorageClass=Auto  FilterContinuousStateAttributes=''  FilterStateMustResolveToSignalObject=off  FilterRTWStateStorageClass=Auto  ParallelPVariant=InternalParameters  IdealPVariant=Disabled  IVariant=InternalParameters  DVariant=InternalParameters  IntegratorVariant=Discrete  SatVariant=Disabled  AWVariant=Passthrough  PCopyVariant=Disabled  TRVariant=Disabled  FdbkBlocksVariant=Forward  IdealPFdbkVariant=Disabled  SatFdbkVariant=Disabled  DerivativeFilterVariant=ForwardEulerFilter  NVariant=InternalParameters  NCopyVariant=Disabled  FilterICVariant=InternalICsFilter  IntegratorICVariant=InternalICs  ExternalResetVariant=Disabled  TRSumVariant=Passthrough  SumFdbkVariant=Disabled  SumVariant=Sum_PID
  Rate Transition : RateTransition  Integrity=off  OutPortSampleTime=t_control
  Rate Transition1 : RateTransition  Integrity=off  OutPortSampleTime=t_control
  Scope3 : Scope  NumInputPorts=2
  Sum3 : Sum  Inputs=-|+
  Terminator{,1..3} (4 alike) : Terminator
  roll,pitch,yaw,climb cmd : Outport
  tag scope: cmd=global
  wires:
  (Y,X,yaw,Z)_est/1 -> Rate Transition/1
  (Y,X,yaw,Z)_cmd/1 -> Rate Transition1/1
  Rate Transition1/1 -> Demux1/1, Sum3/2, [cmd]
  Rate Transition/1 -> Sum3/1
  Demux/2 -> Scope3/2, PID Controller1/1
  Gain1/1 -> Mux/2
  PID Controller4/1 -> Gain/1
  Sum3/1 -> Demux/1
  PID Controller1/1 -> Gain1/1
  Mux/1 -> roll,pitch,yaw,climb cmd/1
  Gain/1 -> Mux/1
  Demux/1 -> Scope3/1, PID Controller4/1
  Demux/3 -> Terminator/1
  Demux/4 -> Terminator1/1
  Demux1/4 -> Mux/4
  Demux1/3 -> Mux/3
  Demux1/1 -> Terminator2/1
  Demux1/2 -> Terminator3/1

== system Sim_Multi/Controller/Controller Structure/Pos//Vel Control/PID Position Controller (yaw and Z are passed though)1 ==
  (Y,X,yaw,Z)_cmd : Inport
  (Y,X,yaw,Z)_est : Inport  Port=2
  Constant : Constant  Value=Kff_1  SampleTime=t_control
  Discrete Derivative : simulink/Discrete/Discrete Derivative  gainval=1.0  ICPrevScaledInput=0.0  OutMin=[]  OutMax=[]  OutDataType=fixdt(1, 16)  OutScaling=2^-10  DoSatur=off
  Discrete-Time Integrator : DiscreteIntegrator  SampleTime=t_control  LimitOutput=on  UpperSaturationLimit=anti_windup_1  LowerSaturationLimit=-1*anti_windup_1  ICPrevOutput=DiscIntNeverNeededParam  ICPrevScaledInput=DiscIntNeverNeededParam
  Gain : Gain  Gain=Kpass_1
  Gain Kd : Subsystem
  Gain Ki : Subsystem
  Gain Kp : Subsystem
  Rate Transition : RateTransition  OutPortSampleTime=t_control
  Rate Transition1 : RateTransition  OutPortSampleTime=t_control
  Sum : Sum  Inputs=+++
  Sum2 : Sum  Inputs=+++
  Sum3 : Sum  Inputs=-|+
  roll,pitch,yaw,climb cmd : Outport
  tag scope: cmd=global
  wires:
  (Y,X,yaw,Z)_est/1 -> Rate Transition/1
  Sum/1 -> roll,pitch,yaw,climb cmd/1
  Gain Ki/1(Out1) -> Discrete-Time Integrator/1
  Discrete-Time Integrator/1 -> Sum2/1
  Gain Kp/1(Out1) -> Sum2/2
  Sum3/1 -> Gain Kp/1(Rate_error), Gain Ki/1(Rate_error)
  (Y,X,yaw,Z)_cmd/1 -> Rate Transition1/1
  Gain Kd/1(Out1) -> Sum/1
  Sum2/1 -> Sum/2
  Constant/1 -> Sum/3
  Discrete Derivative/1 -> Gain Kd/1(Rate_error)
  Rate Transition1/1 -> [cmd], Gain/1, Sum3/2
  Rate Transition/1 -> Discrete Derivative/1, Sum3/1
  Gain/1 -> Sum2/3

== system Sim_Multi/Plant/6DOF model/Calculate omega_dot/Cross Product omega x (J * omega) ==
  omega : Inport
  J * omega : Inport  Port=2
  Subsystem : Subsystem
  Subsystem1 : Subsystem
  Sum : Sum  Inputs=+|-
  omega x (J * omega) : Outport
  wires:
  Sum/1 -> omega x (J * omega)/1
  omega/1 -> Subsystem1/1(u), Subsystem/1(u)
  J * omega/1 -> Subsystem/2(v), Subsystem1/2(v)
  Subsystem/1(Positive elements) -> Sum/1
  Subsystem1/1(Negative elements) -> Sum/2

== system Sim_Multi/Plant/6DOF model/Calculate omega_dot/Subsystem ==
  omega : Inport
  J : Inport  Port=2
  Product : Product  Multiplication=Matrix(*)
  Reshape : Reshape  OutputDimensionality=Column vector (2-D)
  Reshape1 : Reshape  OutputDimensionality=Column vector (2-D)
  J * omega : Outport
  wires:
  Reshape1/1 -> J * omega/1
  Product/1 -> Reshape1/1
  J/1 -> Product/1
  Reshape/1 -> Product/2
  omega/1 -> Reshape/1

== system Sim_Multi/Plant/6DOF model/Quat Strapdown Eq./Cross Product ==
  u : Inport
  v : Inport  Port=2
  Subsystem : Subsystem
  Subsystem1 : Subsystem
  Sum : Sum  Inputs=+|-
  u x v : Outport
  wires:
  Sum/1 -> u x v/1
  u/1 -> Subsystem1/1(u), Subsystem/1(u)
  v/1 -> Subsystem1/2(v), Subsystem/2(v)
  Subsystem/1(Positive elements) -> Sum/1
  Subsystem1/1(Negative elements) -> Sum/2

== system Sim_Multi/Plant/6DOF model/Quat Strapdown Eq./Dot product ==
  u : Inport
  v : Inport  Port=2
  Product : Product  Multiplication=Matrix(*)  RndMeth=Zero
  Reshape : Reshape  OutputDimensionality=Column vector (2-D)
  Reshape1 : Reshape  OutputDimensionality=Column vector (2-D)
  transpose : Math  Operator=transpose  SaturateOnIntegerOverflow=on
  u.v : Outport
  wires:
  v/1 -> Reshape1/1
  u/1 -> Reshape/1
  Reshape/1 -> transpose/1
  transpose/1 -> Product/1
  Reshape1/1 -> Product/2
  Product/1 -> u.v/1

== system Sim_Multi/Plant/6DOF model/Quat Strapdown Eq./Normalize ==
  Input : Inport
  Divide : Product  Inputs=*/
  norm : Subsystem
  Output : Outport
  wires:
  Input/1 -> Divide/1, norm/1(u)
  norm/1(||u||) -> Divide/2
  Divide/1 -> Output/1

== system Sim_Multi/Plant/6DOF model/Quat to Rotation Matrix/Subsystem ==
  q : Inport
  Add : Sum  Inputs=++--
  Demux : Demux
  Product{,2..4} (4 alike) : Product
  C_11 : Outport
  wires:
  Product2/1 -> Add/2
  Product4/1 -> Add/4
  Add/1 -> C_11/1
  Demux/2 -> Product2/2, Product2/1
  Product3/1 -> Add/3
  Demux/3 -> Product3/2, Product3/1
  Demux/1 -> Product/2, Product/1
  q/1 -> Demux/1
  Product/1 -> Add/1
  Demux/4 -> Product4/2, Product4/1

== system Sim_Multi/Plant/6DOF model/Quat to Rotation Matrix/Subsystem1 ==
  q : Inport
  Add : Sum  Inputs=+-+-
  Demux : Demux
  Product{,2..4} (4 alike) : Product
  C_22 : Outport
  wires:
  Product2/1 -> Add/2
  Product4/1 -> Add/4
  Add/1 -> C_22/1
  Demux/2 -> Product2/2, Product2/1
  Product3/1 -> Add/3
  Demux/3 -> Product3/2, Product3/1
  Demux/1 -> Product/2, Product/1
  q/1 -> Demux/1
  Product/1 -> Add/1
  Demux/4 -> Product4/2, Product4/1

== system Sim_Multi/Plant/6DOF model/Quat to Rotation Matrix/Subsystem2 ==
  q : Inport
  Add : Sum  Inputs=+--+
  Demux : Demux
  Product{,2..4} (4 alike) : Product
  C_33 : Outport
  wires:
  Product2/1 -> Add/2
  Product4/1 -> Add/4
  Add/1 -> C_33/1
  Demux/2 -> Product2/2, Product2/1
  Product3/1 -> Add/3
  Demux/3 -> Product3/2, Product3/1
  Demux/1 -> Product/2, Product/1
  q/1 -> Demux/1
  Product/1 -> Add/1
  Demux/4 -> Product4/2, Product4/1

== system Sim_Multi/Plant/6DOF model/Quat to Rotation Matrix/Subsystem3 ==
  q : Inport
  Add : Sum
  Demux : Demux
  Gain : Gain  Gain=2
  Product : Product
  Product2 : Product
  C_12 : Outport
  wires:
  Add/1 -> Gain/1
  q/1 -> Demux/1
  Demux/2 -> Product/1
  Demux/3 -> Product/2
  Demux/1 -> Product2/1
  Demux/4 -> Product2/2
  Product/1 -> Add/1
  Product2/1 -> Add/2
  Gain/1 -> C_12/1

== system Sim_Multi/Plant/6DOF model/Quat to Rotation Matrix/Subsystem4 ==
  q : Inport
  Add : Sum  Inputs=+-
  Demux : Demux
  Gain : Gain  Gain=2
  Product : Product
  Product2 : Product
  C_13 : Outport
  wires:
  Add/1 -> Gain/1
  q/1 -> Demux/1
  Product/1 -> Add/1
  Product2/1 -> Add/2
  Gain/1 -> C_13/1
  Demux/2 -> Product/1
  Demux/4 -> Product/2
  Demux/1 -> Product2/1
  Demux/3 -> Product2/2

== system Sim_Multi/Plant/6DOF model/Quat to Rotation Matrix/Subsystem5 ==
  q : Inport
  Add : Sum  Inputs=+-
  Demux : Demux
  Gain : Gain  Gain=2
  Product : Product
  Product2 : Product
  C_21 : Outport
  wires:
  Add/1 -> Gain/1
  q/1 -> Demux/1
  Product/1 -> Add/1
  Product2/1 -> Add/2
  Gain/1 -> C_21/1
  Demux/2 -> Product/1
  Demux/3 -> Product/2
  Demux/1 -> Product2/1
  Demux/4 -> Product2/2

== system Sim_Multi/Plant/6DOF model/Quat to Rotation Matrix/Subsystem6 ==
  q : Inport
  Add : Sum
  Demux : Demux
  Gain : Gain  Gain=2
  Product : Product
  Product2 : Product
  C_23 : Outport
  wires:
  Add/1 -> Gain/1
  q/1 -> Demux/1
  Product/1 -> Add/1
  Product2/1 -> Add/2
  Gain/1 -> C_23/1
  Demux/3 -> Product/1
  Demux/4 -> Product/2
  Demux/1 -> Product2/1
  Demux/2 -> Product2/2

== system Sim_Multi/Plant/6DOF model/Quat to Rotation Matrix/Subsystem7 ==
  q : Inport
  Add : Sum
  Demux : Demux
  Gain : Gain  Gain=2
  Product : Product
  Product2 : Product
  C_31 : Outport
  wires:
  Add/1 -> Gain/1
  q/1 -> Demux/1
  Product/1 -> Add/1
  Product2/1 -> Add/2
  Gain/1 -> C_31/1
  Demux/2 -> Product/1
  Demux/4 -> Product/2
  Demux/1 -> Product2/1
  Demux/3 -> Product2/2

== system Sim_Multi/Plant/6DOF model/Quat to Rotation Matrix/Subsystem8 ==
  q : Inport
  Add : Sum  Inputs=+-
  Demux : Demux
  Gain : Gain  Gain=2
  Product : Product
  Product2 : Product
  C_32 : Outport
  wires:
  Add/1 -> Gain/1
  q/1 -> Demux/1
  Product/1 -> Add/1
  Product2/1 -> Add/2
  Gain/1 -> C_32/1
  Demux/3 -> Product/1
  Demux/4 -> Product/2
  Demux/1 -> Product2/1
  Demux/2 -> Product2/2

== system Sim_Multi/Plant/6DOF model/Quat to Rotation Matrix/Subsystem9 ==
  C_11 : Inport  PortDimensions=1
  C_12 : Inport  Port=2  PortDimensions=1
  C_13 : Inport  Port=3  PortDimensions=1
  C_21 : Inport  Port=4  PortDimensions=1
  C_22 : Inport  Port=5  PortDimensions=1
  C_23 : Inport  Port=6  PortDimensions=1
  C_31 : Inport  Port=7  PortDimensions=1
  C_32 : Inport  Port=8  PortDimensions=1
  C_33 : Inport  Port=9  PortDimensions=1
  Reshape (9) to [3x3] column-major : Reshape  OutputDimensionality=Customize  OutputDimensions=[3,3]
  Vector Concatenate : Concatenate  NumInputs=9
  DCM_ib : Outport
  wires:
  C_33/1 -> Vector Concatenate/9
  C_22/1 -> Vector Concatenate/5
  Reshape (9) to [3x3] column-major/1 -> DCM_ib/1
  C_11/1 -> Vector Concatenate/1
  Vector Concatenate/1 -> Reshape (9) to [3x3] column-major/1
  C_32/1 -> Vector Concatenate/6
  C_31/1 -> Vector Concatenate/3
  C_21/1 -> Vector Concatenate/2
  C_13/1 -> Vector Concatenate/7
  C_12/1 -> Vector Concatenate/4
  C_23/1 -> Vector Concatenate/8

== system Sim_Multi/Plant/6DOF model/omega x V_b/Subsystem ==
  u : Inport
  v : Inport  Port=2
  Demux : Demux  Outputs=3
  Demux1 : Demux  Outputs=3
  Mux : Mux  Inputs=3
  Product : Product
  Product1 : Product
  Product2 : Product
  Positive elements : Outport
  wires:
  Mux/1 -> Positive elements/1
  v/1 -> Demux1/1
  u/1 -> Demux/1
  Demux/2 -> Product/1
  Demux1/3 -> Product/2
  Demux/3 -> Product1/1
  Demux1/1 -> Product1/2
  Demux/1 -> Product2/1
  Demux1/2 -> Product2/2
  Product/1 -> Mux/1  "u2*v3"
  Product1/1 -> Mux/2  "u3*v1"
  Product2/1 -> Mux/3  "u1*v2"

== system Sim_Multi/Plant/6DOF model/omega x V_b/Subsystem1 ==
  u : Inport
  v : Inport  Port=2
  Demux : Demux  Outputs=3
  Demux1 : Demux  Outputs=3
  Mux : Mux  Inputs=3
  Product : Product
  Product1 : Product
  Product2 : Product
  Negative elements : Outport
  wires:
  Mux/1 -> Negative elements/1
  v/1 -> Demux1/1
  u/1 -> Demux/1
  Product/1 -> Mux/1  "u3*v2"
  Product1/1 -> Mux/2  "u1*v3"
  Product2/1 -> Mux/3  "u2*v1"
  Demux/3 -> Product/1
  Demux1/2 -> Product/2
  Demux/1 -> Product1/1
  Demux1/3 -> Product1/2
  Demux/2 -> Product2/1
  Demux1/1 -> Product2/2

== system Sim_Multi/Plant/Force//Moment computation/Compute aerodynamic drag of the airframe in Body axes/Aerodynamic drag force ==
  note: This block computes the surface area of the airframe that is visible in the direction of the airspeed.
      | Drag force is computed by the standard drag equation: 1/2*rho*u^2*C_D*A
  Airspeed (Body axes) : Inport
  Surface_params : Inport  Port=2
  If : If  IfExpression=u1 == 0
  Merge : Merge
  Nonzero airspeed : Subsystem  TreatAsAtomicUnit=on
  Zero airspeed : Subsystem  TreatAsAtomicUnit=on
  norm : Subsystem
  Drag force (Body axes) : Outport
  wires:
  If/1 -> Zero airspeed/Action
  Zero airspeed/1(Drag force) -> Merge/1
  Nonzero airspeed/1(Drag force) -> Merge/2
  If/2 -> Nonzero airspeed/Action
  Airspeed (Body axes)/1 -> norm/1(u), Nonzero airspeed/1(Airspeed (Body)), Zero airspeed/1(Airspeed)
  norm/1(||u||) -> If/1  "Airspeed magnitude"
  Merge/1 -> Drag force (Body axes)/1  "Force against direction of motion due to aerodynamic drag"
  Surface_params/1 -> Nonzero airspeed/2(Surface_params), Zero airspeed/2(Surface_params)

== system Sim_Multi/Plant/Force//Moment computation/Compute aerodynamic drag of the airframe in Body axes/Total airspeed (Body axes) ==
  V_b : Inport
  DCM_ib : Inport  Port=2
  Wind_i : Inport  Port=3
  Inertial to Body : Subsystem
  Reshape : Reshape  OutputDimensionality=Column vector (2-D)
  Sum1 : Sum  Inputs=|+-
  Airspeed (Body) : Outport
  wires:
  DCM_ib/1 -> Inertial to Body/1(DCM_ib)
  Wind_i/1 -> Inertial to Body/2(Wind_i)
  Inertial to Body/1(Wind_b) -> Sum1/2  "Wind velocity (Body axes)"
  Reshape/1 -> Sum1/1
  V_b/1 -> Reshape/1
  Sum1/1 -> Airspeed (Body)/1  "True airspeed (Body axes)"

== system Sim_Multi/Plant/Force//Moment computation/Forces and moments generated by spinning propellers/For Each Subsystem ==
  note: This subsystem computes all the forces and moments generated by each of the actuators.
      |
      | That includes dynamic thrust, blade flapping effects, gyroscopic moments, and others.
      | All forces and moments are computed as acting on the real center of gravity of the airframe,
      | which might change during the simulation due to failure cases or the dropping of cargo.
      |
      | Outputs are the total force and moment vectors for each one of the motors.
  RPM_commands : Inport  Partition=on  PartitionDimension=1  PartitionWidth=1  PartitionOffset=0
  Body_rates : Inport  Port=2
  Airspeed (Body) : Inport  Port=3
  MotorMatrix_real : Inport  Port=4  Partition=on  PartitionDimension=1  PartitionWidth=1  PartitionOffset=0
  CoG_real : Inport  Port=5
  6 DOF : Inport  Port=6
  Actuator dynamics : Subsystem
  Cross Product : Subsystem
  For Each : ForEach  DisableCoverage=on
  Leverarm vector from real CoG to each propeller (Body axes) : Subsystem
  Rate Transition : RateTransition  OutPortSampleTime=t_sim
  Sum1 : Sum  Inputs=|++
  Thrust/moment vector for each propeller (Body axes) : Subsystem
  Motor_force : Outport  ConcatenationDimension=2
  Motor_moment : Outport  Port=2  ConcatenationDimension=2
  RPM_motor : Outport  Port=3  ConcatenationDimension=2
  wires:
  Leverarm vector from real CoG to each propeller (Body axes)/1(Prop_vector) -> Cross Product/1(r), Thrust/moment vector for each propeller (Body axes)/1(Prop_vector)  "Leverarm vector from real CoG to propeller (Body axes)"
  MotorMatrix_real/1 -> Leverarm vector from real CoG to each propeller (Body axes)/1(MotorMatrix_real), Thrust/moment vector for each propeller (Body axes)/4(MotorMatrix_real), Actuator dynamics/1(MotorMatrix_real)
  Thrust/moment vector for each propeller (Body axes)/1(Thrust_vector (Body axes)) -> Motor_force/1  "Thrust force vector for each motor (Body axes)"
  Thrust/moment vector for each propeller (Body axes)/2(Motor_moments (Body axes)) -> Motor_moment/1  "Moment vector for each motor (Body axes)"
  RPM_commands/1 -> Rate Transition/1
  Body_rates/1 -> Thrust/moment vector for each propeller (Body axes)/3(Body_rates), Cross Product/2(omega)
  CoG_real/1 -> Leverarm vector from real CoG to each propeller (Body axes)/2(CoG_real)
  Cross Product/1(omega x r) -> Sum1/1  "Linear velocity at prop due to body angular rates (Body axes)"
  Airspeed (Body)/1 -> Sum1/2  "True linear velocity of airframe (including wind) (Body axes)"
  Sum1/1 -> Thrust/moment vector for each propeller (Body axes)/2(True airspeed)  "Total linear velocity at prop (Body axes)"
  Actuator dynamics/1(RPM_motor) -> RPM_motor/1, Thrust/moment vector for each propeller (Body axes)/5(RPM_motor)  "Actual motor RPM"
  Rate Transition/1 -> Actuator dynamics/2(RPM_command)
  6 DOF/1 -> Thrust/moment vector for each propeller (Body axes)/6(6 DOF)

== system Sim_Multi/Plant/Force//Moment computation/Forces and moments generated by spinning propellers/Total airspeed (Body axes) ==
  V_b : Inport
  DCM_ib : Inport  Port=2
  Wind_i : Inport  Port=3
  Inertial to Body : Subsystem
  Reshape : Reshape  OutputDimensionality=Column vector (2-D)
  Sum1 : Sum  Inputs=|+-
  Airspeed (Body) : Outport
  wires:
  DCM_ib/1 -> Inertial to Body/1(DCM_ib)
  Wind_i/1 -> Inertial to Body/2(Wind_i)
  Inertial to Body/1(Wind_b) -> Sum1/2  "Wind velocity (Body axes)"
  Sum1/1 -> Airspeed (Body)/1  "True airspeed (Body axes)"
  Reshape/1 -> Sum1/1
  V_b/1 -> Reshape/1

== system Sim_Multi/State Estimation, Sensors, Noise/State estimation/Normalize/norm ==
  u : Inport
  Complex to Real-Imag : ComplexToRealImag  Output=Real
  Sqrt : Sqrt  SaturateOnIntegerOverflow=on
  dot_product : Subsystem
  ||u|| : Outport
  wires:
  u/1 -> dot_product/1(u), dot_product/2(v)
  dot_product/1(u.v) -> Sqrt/1
  Sqrt/1 -> Complex to Real-Imag/1
  Complex to Real-Imag/1 -> ||u||/1

== system Sim_Multi/State Estimation, Sensors, Noise/State estimation/Normalize1/norm ==
  u : Inport
  Complex to Real-Imag : ComplexToRealImag  Output=Real
  Sqrt : Sqrt  SaturateOnIntegerOverflow=on
  dot_product : Subsystem
  ||u|| : Outport
  wires:
  u/1 -> dot_product/1(u), dot_product/2(v)
  dot_product/1(u.v) -> Sqrt/1
  Sqrt/1 -> Complex to Real-Imag/1
  Complex to Real-Imag/1 -> ||u||/1

== system Sim_Multi/Controller/Controller Structure/Pos//Vel Control/PI Rate controller1/Cross Product ==
  u : Inport
  v : Inport  Port=2
  Subsystem : Subsystem
  Subsystem1 : Subsystem
  Sum : Sum  Inputs=+|-
  u x v : Outport
  wires:
  Sum/1 -> u x v/1
  u/1 -> Subsystem1/1(u), Subsystem/1(u)
  v/1 -> Subsystem1/2(v), Subsystem/2(v)
  Subsystem/1(Positive elements) -> Sum/1
  Subsystem1/1(Negative elements) -> Sum/2
